simulink model "evaluate_state_feedback"  (R2020b)
settings: Solver=VariableStepAuto  StartTime=0.0  StopTime=1100  RelTol=1e-3
settings Model: Creator=sharm  LastModifiedBy=Abhijit

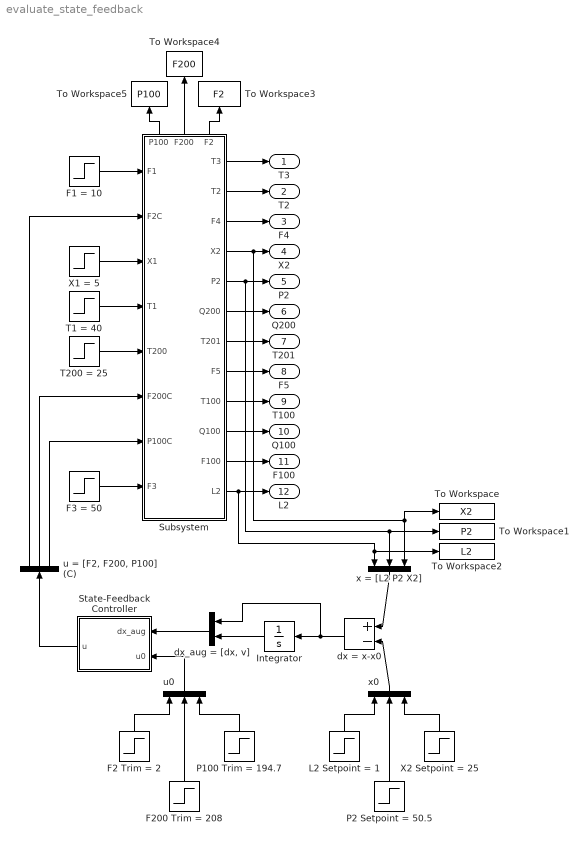
== system evaluate_state_feedback ==
  F1 = 10 : Step  Time=0  After=10  SampleTime=0
  F2 Trim = 2 : Step  Time=0  After=2  SampleTime=0
  F200 Trim = 208 : Step  Time=0  After=208  SampleTime=0
  F3 = 50 : Step  Time=0  After=50  SampleTime=0
  Integrator : Integrator
  L2 Setpoint = 1 : Step  Time=0  SampleTime=0
  P100 Trim = 194.7 : Step  Time=0  After=194.7  SampleTime=0
  P2 Setpoint = 50.5 : Step  Time=0  After=50.5  SampleTime=0
  State-Feedback Controller : MATLAB Function  TreatAsAtomicUnit=on
  Subsystem : Subsystem
      settings: PortSchema="{\"entries\":[{\"content\":{\"sides\":[{\"content\":{\"connectorIds\":[\"In1\",\"In2\",\"In3\",\"In4\",\"In5\",\"In6\",\"In7\",\"In8\"]},\"type\":\"ConnectorPlacement.EquallySpacedRectSide\",\"uuid\":\"f9a1b81a-b99e-4913-8393-08c2fe40246f\"},{\"content\":{\"connectorIds\":[\"Out1\",\"Out2\",\"Out3\",\"Out4\",\"Out5\",\"Out6\",\"Out7\",\"Out8\",\"Out9\",\"Out10\",\"Out11\",\"Out12\"],\"side\":\"RIGHT\"},\"type\":\"ConnectorPlacement.EquallySpacedRectSide\",\"uuid\":\"82085886-3e26-4210-9d85-7a5d2324261f\"},{\"content\":{\"connectorIds\":[\"Out13\",\"Out14\",\"Out15\"],\"side\":\"TOP\"},\"type\":\"ConnectorPlacement.EquallySpacedRectSide\",\"uuid\":\"41f001c5-6b1a-48ec-bf6d-aea194c7eab1\"},{\"content\":{\"connectorIds\":[],\"side\":\"HIDDEN\"},\"type\":\"ConnectorPlacement.EquallySpacedRectSide\",\"uuid\":\"d940c032-0398-4951-9103-a0a10b191a5d\"}]},\"type\":\"ConnectorPlacement.EquallySpacedConnector\",\"uuid\":\"422c0c1a-3552-44cb-aa63-012fdb829581\"}],\"packageUris\":[\"http://schema.mathworks.com/mf0/Connector/R2020b\"],\"version\":\"1.0\"}"
  T1 = 40 : Step  Time=0  After=40  SampleTime=0
  T200 = 25 : Step  Time=0  After=25  SampleTime=0
  To Workspace : ToWorkspace  VariableName=X2  SaveFormat=Timeseries  SampleTime=-1
  To Workspace1 : ToWorkspace  VariableName=P2  SaveFormat=Timeseries  SampleTime=-1
  To Workspace2 : ToWorkspace  VariableName=L2  SaveFormat=Timeseries  SampleTime=-1
  To Workspace3 : ToWorkspace  VariableName=F2  SaveFormat=Timeseries  SampleTime=-1
  To Workspace4 : ToWorkspace  VariableName=F200  SaveFormat=Timeseries  SampleTime=-1
  To Workspace5 : ToWorkspace  VariableName=P100  SaveFormat=Timeseries  SampleTime=-1
  X1 = 5 : Step  Time=0  After=5  SampleTime=0
  X2 Setpoint = 25 : Step  Time=0  After=25  SampleTime=0
  dx = x-x0 : Sum  Inputs=+-
  "dx_aug = [dx, v]" : Mux  Inputs=2
  "u = [F2, F200, P100] (C)" : Demux  Outputs=3
  u0 : Mux  Inputs=3
  x = [L2 P2 X2] : Mux  Inputs=3
  x0 : Mux  Inputs=3
  T3 : Outport
  T2 : Outport  Port=2
  F4 : Outport  Port=3
  X2 : Outport  Port=4
  P2 : Outport  Port=5
  Q200 : Outport  Port=6
  T201 : Outport  Port=7
  F5 : Outport  Port=8
  T100 : Outport  Port=9
  Q100 : Outport  Port=10
  F100 : Outport  Port=11
  L2 : Outport  Port=12
  wires:
  F1 = 10/1 -> Subsystem/1(F1)
  X1 = 5/1 -> Subsystem/3(X1)
  T1 = 40/1 -> Subsystem/4(T1)
  T200 = 25/1 -> Subsystem/5(T200)
  F3 = 50/1 -> Subsystem/8(F3)
  Subsystem/1(T3) -> T3/1
  Subsystem/2(T2) -> T2/1
  Subsystem/3(F4) -> F4/1
  Subsystem/4(X2) -> To Workspace/1, x = [L2 P2 X2]/3, X2/1
  Subsystem/5(P2) -> x = [L2 P2 X2]/2, To Workspace1/1, P2/1
  Subsystem/6(Q200) -> Q200/1
  Subsystem/7(T201) -> T201/1
  Subsystem/8(F5) -> F5/1
  Subsystem/9(T100) -> T100/1
  Subsystem/10(Q100) -> Q100/1
  Subsystem/11(F100) -> F100/1
  Subsystem/12(L2) -> To Workspace2/1, x = [L2 P2 X2]/1, L2/1
  State-Feedback Controller/1(u) -> "u = [F2, F200, P100] (C)"/1
  "u = [F2, F200, P100] (C)"/1 -> Subsystem/2(F2C)
  "u = [F2, F200, P100] (C)"/2 -> Subsystem/6(F200C)
  "u = [F2, F200, P100] (C)"/3 -> Subsystem/7(P100C)
  u0/1 -> State-Feedback Controller/2(u0)
  F2 Trim = 2/1 -> u0/1
  P100 Trim = 194.7/1 -> u0/3
  F200 Trim = 208/1 -> u0/2
  X2 Setpoint = 25/1 -> x0/3
  P2 Setpoint = 50.5/1 -> x0/2
  L2 Setpoint = 1/1 -> x0/1
  x0/1 -> dx = x-x0/2
  x = [L2 P2 X2]/1 -> dx = x-x0/1
  dx = x-x0/1 -> "dx_aug = [dx, v]"/1, Integrator/1
  Integrator/1 -> "dx_aug = [dx, v]"/2
  "dx_aug = [dx, v]"/1 -> State-Feedback Controller/1(dx_aug)
  Subsystem/15(F2) -> To Workspace3/1
  Subsystem/13(P100) -> To Workspace5/1
  Subsystem/14(F200) -> To Workspace4/1

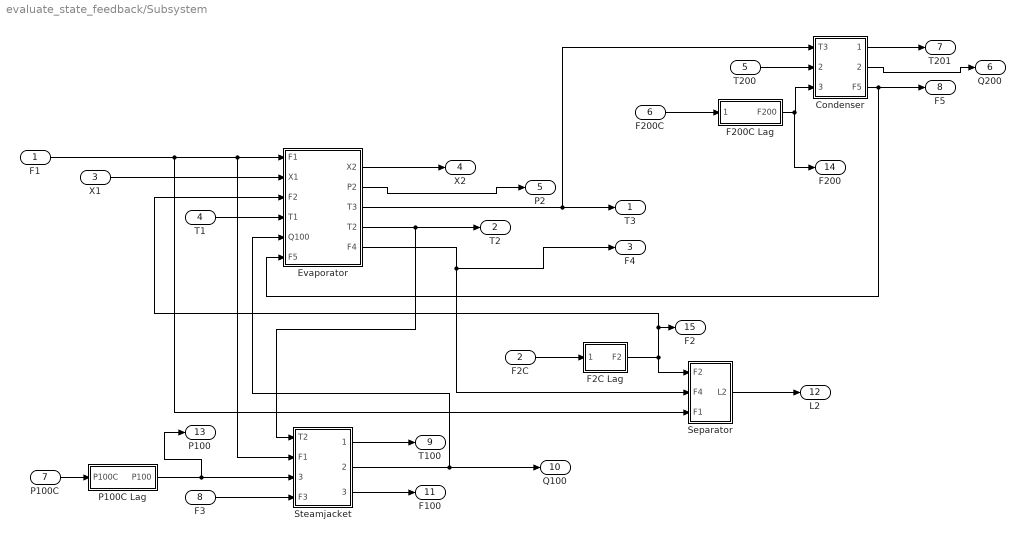
== system evaluate_state_feedback/Subsystem ==
  F1 : Inport
  F2C : Inport  Port=2
  X1 : Inport  Port=3
  T1 : Inport  Port=4
  T200 : Inport  Port=5
  F200C : Inport  Port=6
  P100C : Inport  Port=7
  F3 : Inport  Port=8
  Condenser : Subsystem
  Evaporator : Subsystem
  F200C Lag : Subsystem
  F2C Lag : Subsystem
  P100C Lag : Subsystem
  Separator : Subsystem
  Steamjacket : Subsystem
  T3 : Outport
  T2 : Outport  Port=2
  F4 : Outport  Port=3
  X2 : Outport  Port=4
  P2 : Outport  Port=5
  Q200 : Outport  Port=6
  T201 : Outport  Port=7
  F5 : Outport  Port=8
  T100 : Outport  Port=9
  Q100 : Outport  Port=10
  F100 : Outport  Port=11
  L2 : Outport  Port=12
  P100 : Outport  Port=13
  F200 : Outport  Port=14
  F2 : Outport  Port=15
  wires:
  X1/1 -> Evaporator/2(X1)
  Condenser/3(F5) -> F5/1, Evaporator/6(F5)
  T200/1 -> Condenser/2(T200)
  Condenser/1(T201) -> T201/1
  Steamjacket/2(Q100) -> Q100/1, Evaporator/5(Q100)
  F1/1 -> Steamjacket/2(F1), Evaporator/1(F1), Separator/3(F1)
  Evaporator/2(P2) -> P2/1
  Evaporator/3(T3) -> T3/1, Condenser/1(T3)
  F2C/1 -> F2C Lag/1(F2C)
  Evaporator/1(X2) -> X2/1
  F2C Lag/1(F2) -> F2/1, Evaporator/3(F2), Separator/1(F2)
  T1/1 -> Evaporator/4(T1)
  Evaporator/5(F4) -> F4/1, Separator/2(F4)
  Steamjacket/3(F100) -> F100/1
  F3/1 -> Steamjacket/4(F3)
  Evaporator/4(T2) -> T2/1, Steamjacket/1(T2)
  Steamjacket/1(T100) -> T100/1
  Condenser/2(Q200) -> Q200/1
  P100C/1 -> P100C Lag/1(P100C)
  F200C Lag/1(F200) -> F200/1, Condenser/3(F200)
  F200C/1 -> F200C Lag/1(F200C)
  Separator/1(L2) -> L2/1
  P100C Lag/1(P100) -> P100/1, Steamjacket/3(P100)

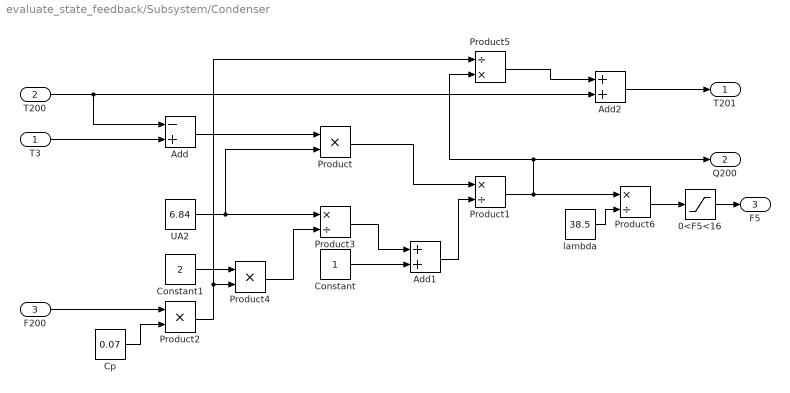
== system evaluate_state_feedback/Subsystem/Condenser ==
  T3 : Inport
  T200 : Inport  Port=2
  F200 : Inport  Port=3
  0<F5<16 : Saturate  UpperLimit=16  LowerLimit=0
  Add : Sum  Inputs=-+
  Add1 : Sum
  Add2 : Sum
  Constant : Constant
  Constant1 : Constant  Value=2
  Cp : Constant  Value=0.07
  Product : Product
  Product1 : Product  Inputs=*/
  Product2 : Product
  Product3 : Product  Inputs=*/
  Product4 : Product
  Product5 : Product  Inputs=/*
  Product6 : Product  Inputs=*/
  UA2 : Constant  Value=6.84
  lambda : Constant  Value=38.5
  T201 : Outport
  Q200 : Outport  Port=2
  F5 : Outport  Port=3
  wires:
  Product1/1 -> Q200/1, Product5/2, Product6/1
  lambda/1 -> Product6/2
  Product5/1 -> Add2/1
  Constant1/1 -> Product4/1
  Product2/1 -> Product5/1, Product4/2
  Constant/1 -> Add1/2
  Add/1 -> Product/1
  Cp/1 -> Product2/2
  Product4/1 -> Product3/2
  T200/1 -> Add2/2, Add/1
  Product/1 -> Product1/1
  Add2/1 -> T201/1
  Product3/1 -> Add1/1
  UA2/1 -> Product3/1, Product/2
  T3/1 -> Add/2
  F200/1 -> Product2/1
  Add1/1 -> Product1/2
  Product6/1 -> 0<F5<16/1
  0<F5<16/1 -> F5/1

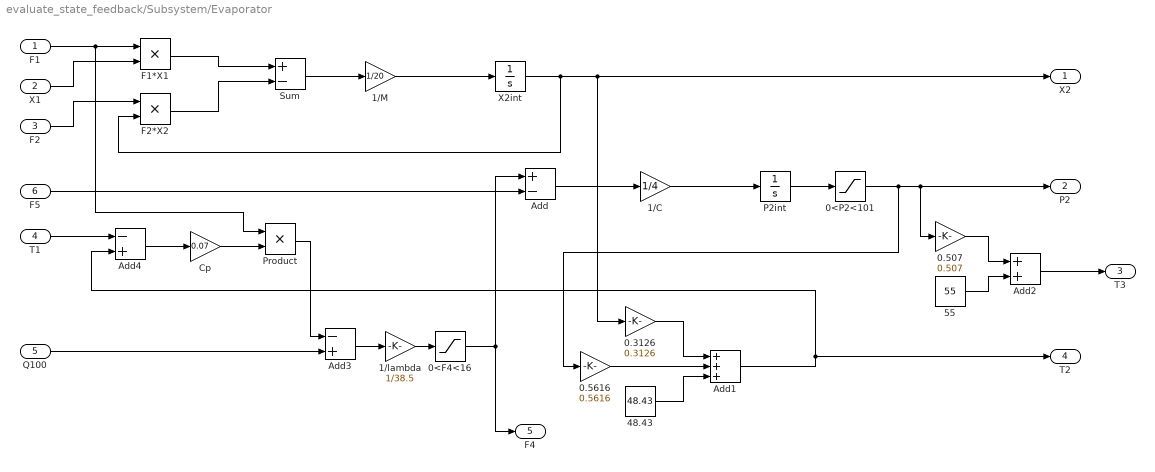
== system evaluate_state_feedback/Subsystem/Evaporator ==
  F1 : Inport
  X1 : Inport  Port=2
  F2 : Inport  Port=3
  T1 : Inport  Port=4
  Q100 : Inport  Port=5
  F5 : Inport  Port=6
  0.3126 : Gain  Gain=0.3126
  0.507 : Gain  Gain=0.507
  0.5616 : Gain  Gain=0.5616
  0<F4<16 : Saturate  UpperLimit=16  LowerLimit=0
  0<P2<101 : Saturate  UpperLimit=101  LowerLimit=0
  1/C : Gain  Gain=1/4
  1/M : Gain  Gain=1/20
  1/lambda : Gain  Gain=1/38.5
  48.43 : Constant  Value=48.43
  55 : Constant  Value=55
  Add : Sum  Inputs=+-
  Add1 : Sum  Inputs=+++
  Add2 : Sum
  Add3 : Sum  Inputs=-+
  Add4 : Sum  Inputs=-+
  Cp : Gain  Gain=0.07
  F1*X1 : Product
  F2*X2 : Product
  P2int : Integrator  InitialCondition=50.5
  Product : Product
  Sum : Sum  Inputs=+-
  X2int : Integrator  InitialCondition=25
  X2 : Outport
  P2 : Outport  Port=2
  T3 : Outport  Port=3
  T2 : Outport  Port=4
  F4 : Outport  Port=5
  wires:
  Product/1 -> Add3/1
  Add4/1 -> Cp/1
  Add1/1 -> T2/1, Add4/2
  Add/1 -> 1/C/1
  F1/1 -> Product/1, F1*X1/1
  Add2/1 -> T3/1
  X2int/1 -> X2/1, 0.3126/1, F2*X2/2
  0.507/1 -> Add2/1
  Cp/1 -> Product/2
  F1*X1/1 -> Sum/1
  0.3126/1 -> Add1/1
  1/C/1 -> P2int/1
  F2/1 -> F2*X2/1
  1/M/1 -> X2int/1
  Sum/1 -> 1/M/1
  48.43/1 -> Add1/3
  F2*X2/1 -> Sum/2
  Add3/1 -> 1/lambda/1
  Q100/1 -> Add3/2
  F5/1 -> Add/2
  55/1 -> Add2/2
  0.5616/1 -> Add1/2
  T1/1 -> Add4/1
  X1/1 -> F1*X1/2
  0<F4<16/1 -> F4/1, Add/1
  1/lambda/1 -> 0<F4<16/1
  P2int/1 -> 0<P2<101/1
  0<P2<101/1 -> 0.5616/1, 0.507/1, P2/1

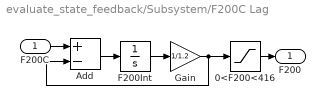
== system evaluate_state_feedback/Subsystem/F200C Lag ==
  F200C : Inport
  0<F200<416 : Saturate  UpperLimit=416  LowerLimit=0
  Add : Sum  Inputs=+-
  F200Int : Integrator  InitialCondition=208
  Gain : Gain  Gain=1/1.2
  F200 : Outport
  wires:
  Gain/1 -> Add/2, 0<F200<416/1
  Add/1 -> F200Int/1
  F200Int/1 -> Gain/1
  F200C/1 -> Add/1
  0<F200<416/1 -> F200/1

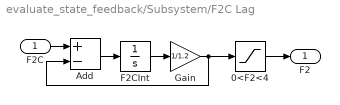
== system evaluate_state_feedback/Subsystem/F2C Lag ==
  F2C : Inport
  0<F2<4 : Saturate  UpperLimit=4  LowerLimit=0
  Add : Sum  Inputs=+-
  F2CInt : Integrator  InitialCondition=2
  Gain : Gain  Gain=1/1.2
  F2 : Outport
  wires:
  Gain/1 -> Add/2, 0<F2<4/1
  Add/1 -> F2CInt/1
  F2CInt/1 -> Gain/1
  F2C/1 -> Add/1
  0<F2<4/1 -> F2/1

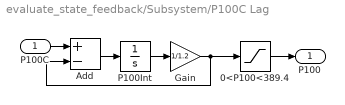
== system evaluate_state_feedback/Subsystem/P100C Lag ==
  P100C : Inport
  0<P100<389.4 : Saturate  UpperLimit=389.4  LowerLimit=0
  Add : Sum  Inputs=+-
  Gain : Gain  Gain=1/1.2
  P100Int : Integrator  InitialCondition=194.7
  P100 : Outport
  wires:
  Gain/1 -> Add/2, 0<P100<389.4/1
  Add/1 -> P100Int/1
  P100Int/1 -> Gain/1
  P100C/1 -> Add/1
  0<P100<389.4/1 -> P100/1

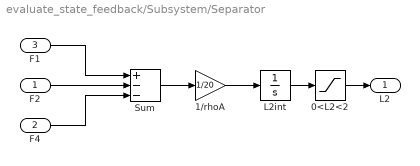
== system evaluate_state_feedback/Subsystem/Separator ==
  F2 : Inport
  F4 : Inport  Port=2
  F1 : Inport  Port=3
  0<L2<2 : Saturate  UpperLimit=2  LowerLimit=0
  1/rhoA : Gain  Gain=1/20
  L2int : Integrator  InitialCondition=1
  Sum : Sum  Inputs=+--
  L2 : Outport
  wires:
  F4/1 -> Sum/3
  1/rhoA/1 -> L2int/1
  Sum/1 -> 1/rhoA/1
  F2/1 -> Sum/2
  F1/1 -> Sum/1
  L2int/1 -> 0<L2<2/1
  0<L2<2/1 -> L2/1

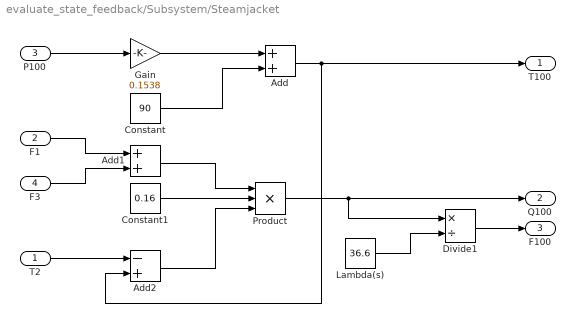
== system evaluate_state_feedback/Subsystem/Steamjacket ==
  T2 : Inport
  F1 : Inport  Port=2
  P100 : Inport  Port=3
  F3 : Inport  Port=4
  Add : Sum
  Add1 : Sum
  Add2 : Sum  Inputs=-+
  Constant : Constant  Value=90
  Constant1 : Constant  Value=0.16
  Divide1 : Product  Inputs=*/
  Gain : Gain  Gain=0.1538
  Lambda(s) : Constant  Value=36.6  VectorParams1D=off
  Product : Product  Inputs=3
  T100 : Outport
  Q100 : Outport  Port=2
  F100 : Outport  Port=3
  wires:
  Add1/1 -> Product/1
  Constant1/1 -> Product/2
  Product/1 -> Q100/1, Divide1/1
  Gain/1 -> Add/1
  Add2/1 -> Product/3
  Lambda(s)/1 -> Divide1/2
  Constant/1 -> Add/2
  Add/1 -> T100/1, Add2/2
  P100/1 -> Gain/1
  T2/1 -> Add2/1
  Divide1/1 -> F100/1
  F3/1 -> Add1/2
  F1/1 -> Add1/1

== matlab function evaluate_state_feedback/State-Feedback Controller ==
  data: dx_aug input; u output; u0 input
function u = fcn(dx_aug, u0)  
    K_L = 1.0e+03 * [
   -0.0000    0.0000   -0.0011   -0.0000    0.0000   -0.0004;
   -4.2105   -0.8234    0.1570   -1.4035   -0.2778    0.0561;
   -0.7895   -0.0039    0.0273   -0.2632   -0.0000    0.0105
   ];
 
    du = -(K_L)*dx_aug;
    u = du + u0;
end
